simulink model "rhpZeros"  (R2015a)
settings: Solver=ode3  StartTime=0.0  StopTime=10.0  FixedStep=1/200  RelTol=1e-3
undefined symbols (not defined in the file or in its folder): Hinf
libraries: PoliArd x9, simulink x3, dspswit3 x1
settings Model: ExtModeTrigDuration=2  Creator=user  LastModifiedBy=user
settings OptimizationCC: OptimizeModelRefInitCode=on  LifeSpan=1
settings DebuggingCC: UnderspecifiedInitializationDetection=Classic  MergeDetectMultiDrivingBlocksExec=none
settings HardwareCC: ProdLargestAtomicInteger=Long  ProdLargestAtomicFloat=Double  ProdEndianess=LittleEndian  ProdHWDeviceType=ARM Compatible->ARM Cortex
settings RTWCC: SystemTargetFile=realtime.tlc  GenerateMakefile=off  TemplateMakefile=realtime.tmf  Description=Run on Target Hardware  RTWVerbose=off
settings ERTTargetCC: CombineOutputUpdateFcns=off  ExtModeTransport=3  ExtModeMexFile=ext_serial_win32_comm_rtt  ExtModeMexArgs=0 1 9600  ERTSrcFileBannerTemplate=realtime_code_template.cgt  ERTHdrFileBannerTemplate=realtime_code_template.cgt  ERTDataSrcFileTemplate=realtime_code_template.cgt  ERTDataHdrFileTemplate=realtime_code_template.cgt  ERTCustomFileTemplate=realtime_file_process.tlc

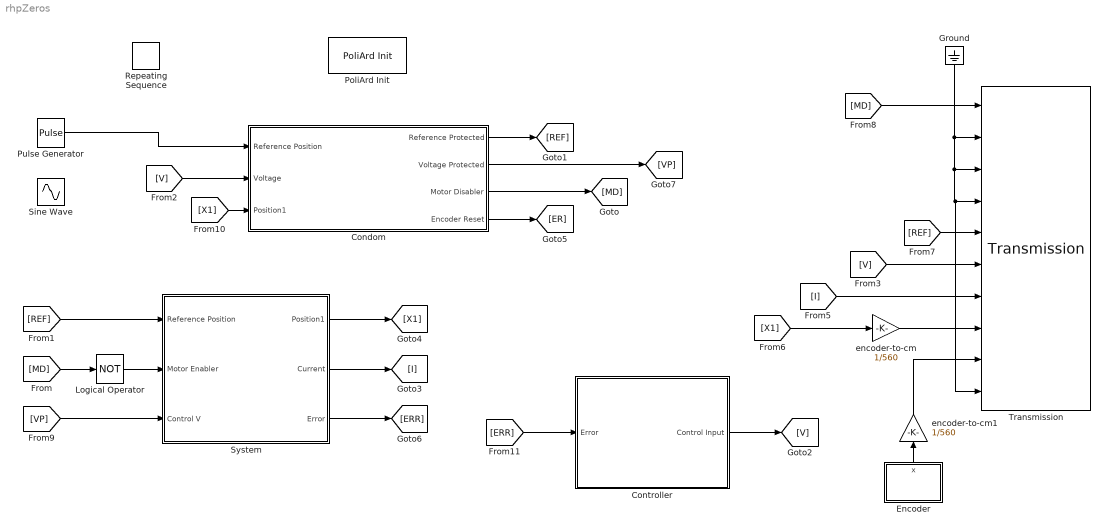
== system rhpZeros ==
  Condom : Subsystem
  Controller : Subsystem
  "Encoder " : Subsystem
  Ground : Ground
  Logical Operator : Logic  Operator=NOT  AllPortsSameDT=off  OutDataTypeStr=boolean
  PoliArd Init : PoliArd/PoliArd Init
  Pulse Generator : DiscretePulseGenerator  PulseType=Time based  Period=10  PulseWidth=50  PhaseDelay=5
  Repeating Sequence : simulink/Sources/Repeating Sequence  rep_seq_t=[0 5]  rep_seq_y=[0 1]
  Sine Wave : Sin  Frequency=2*pi*1  SampleTime=0
  "System " : Subsystem
  Transmission : PoliArd/Transmission  sample_freq=200  sig_to_send=6
  encoder-to-cm : Gain  Gain=1/560
  encoder-to-cm1 : Gain  Gain=1/560
  wires:
  Logical Operator/1 -> "System "/2(Motor Enabler)
  [MD] -> Logical Operator/1
  Condom/1(Reference Protected) -> [REF]
  [REF] -> "System "/1(Reference Position)
  "System "/2(Current) -> [I]
  [V] -> Condom/2(Voltage)
  [V] -> Transmission/6
  [I] -> Transmission/7
  "System "/1(Position1) -> [X1]
  [X1] -> encoder-to-cm/1
  [REF] -> Transmission/5
  [MD] -> Transmission/1
  [VP] -> "System "/3(Control V)
  [X1] -> Condom/3(Position1)
  encoder-to-cm/1 -> Transmission/8
  Controller/1(Control Input) -> [V]
  "System "/3(Error) -> [ERR]
  [ERR] -> Controller/1(Error)
  Condom/2("Voltage Protected ") -> [VP]
  Condom/3(Motor Disabler) -> [MD]
  Condom/4(Encoder Reset) -> [ER]
  Ground/1 -> Transmission/10, Transmission/4, Transmission/3, Transmission/2
  Pulse Generator/1 -> Condom/1(Reference Position)
  "Encoder "/1(x) -> encoder-to-cm1/1
  encoder-to-cm1/1 -> Transmission/9

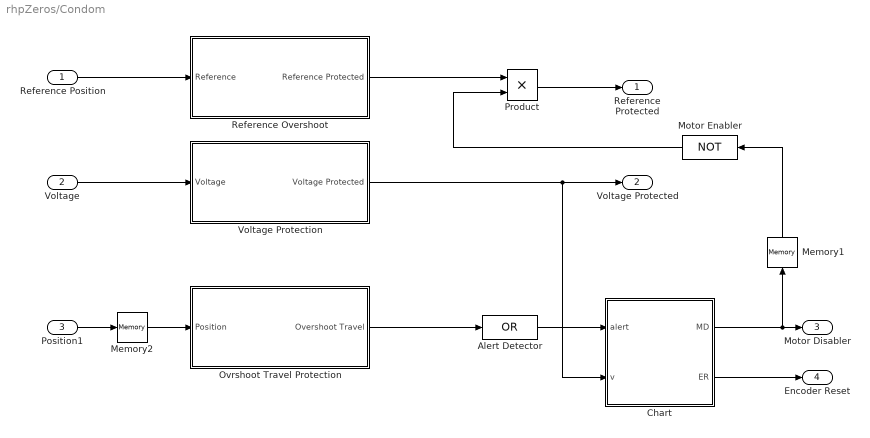
== system rhpZeros/Condom ==
  Reference Position : Inport
  Voltage : Inport  Port=2
  Position1 : Inport  Port=3
  Alert Detector : Logic  Operator=OR  Inputs=1  AllPortsSameDT=off  OutDataTypeStr=boolean
  Chart : Stateflow chart  TreatAsAtomicUnit=on
  Memory1 : Memory
  Memory2 : Memory
  Motor Enabler : Logic  Operator=NOT  Inputs=1  AllPortsSameDT=off  OutDataTypeStr=boolean
  Ovrshoot Travel Protection : Subsystem
  Product : Product
  Reference Overshoot : Subsystem
  Voltage Protection : Subsystem
  Reference Protected : Outport
  "Voltage Protected " : Outport  Port=2
  Motor Disabler : Outport  Port=3
  Encoder Reset : Outport  Port=4
  wires:
  Reference Position/1 -> Reference Overshoot/1("Reference ")
  Memory2/1 -> Ovrshoot Travel Protection/1("Position ")
  Position1/1 -> Memory2/1
  Ovrshoot Travel Protection/1(Overshoot Travel) -> Alert Detector/1
  Alert Detector/1 -> Chart/1(alert)
  Chart/1(MD) -> Motor Disabler/1, Memory1/1
  Chart/2(ER) -> Encoder Reset/1
  Voltage/1 -> Voltage Protection/1("Voltage ")
  Voltage Protection/1(Voltage Protected) -> Chart/2(v), "Voltage Protected "/1
  Product/1 -> Reference Protected/1
  Reference Overshoot/1(Reference Protected) -> Product/1
  Motor Enabler/1 -> Product/2
  Memory1/1 -> Motor Enabler/1

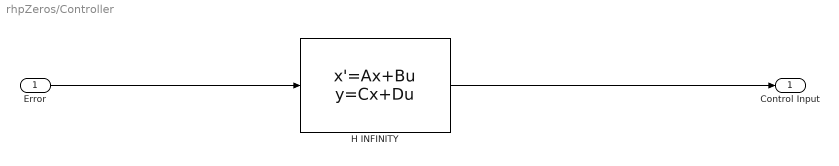
== system rhpZeros/Controller ==
  Error : Inport
  H INFINITY : StateSpace  A=Hinf.A  B=Hinf.B  C=Hinf.C  D=Hinf.D  X0=0
  Control Input : Outport
  wires:
  Error/1 -> H INFINITY/1
  H INFINITY/1 -> Control Input/1

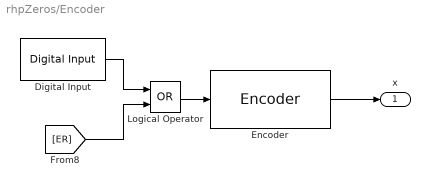
== system rhpZeros/Encoder  ==
  Digital Input : PoliArd/Digital Input  DI_pin=2  DIsample=1/200
  Encoder : PoliArd/Encoder  EncoderID=4  dt_enc=1/200
  Logical Operator : Logic  Operator=OR  AllPortsSameDT=off  OutDataTypeStr=boolean
  x : Outport
  wires:
  Encoder/1 -> x/1
  Digital Input/1 -> Logical Operator/1
  [ER] -> Logical Operator/2
  Logical Operator/1 -> Encoder/1

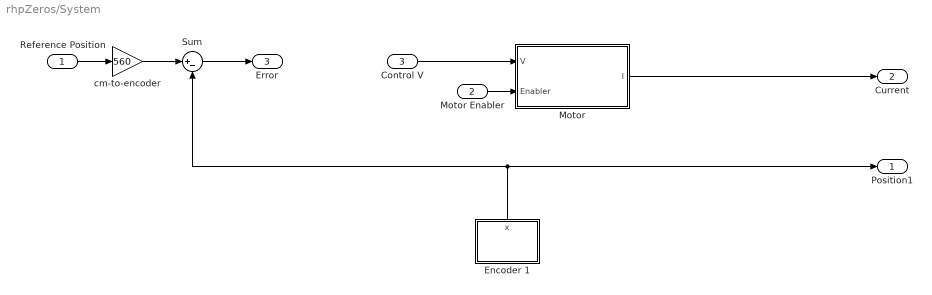
== system rhpZeros/System  ==
  Reference Position : Inport
  Motor Enabler : Inport  Port=2
  Control V : Inport  Port=3
  "Encoder 1 " : Subsystem
  Motor : Subsystem
  Sum : Sum  Inputs=|+-
  cm-to-encoder : Gain  Gain=560
  Position1 : Outport
  Current : Outport  Port=2
  Error : Outport  Port=3
  wires:
  cm-to-encoder/1 -> Sum/1
  Motor/1(I) -> Current/1
  Sum/1 -> Error/1
  Reference Position/1 -> cm-to-encoder/1
  Motor Enabler/1 -> Motor/2(Enabler)
  Control V/1 -> Motor/1(V)
  "Encoder 1 "/1(x) -> Position1/1, Sum/2

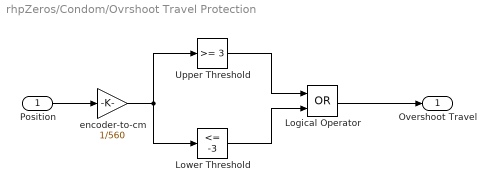
== system rhpZeros/Condom/Ovrshoot Travel Protection ==
  "Position " : Inport
  Logical Operator : Logic  Operator=OR  AllPortsSameDT=off  OutDataTypeStr=boolean
  Lower Threshold : simulink/Logic and Bit Operations/Compare To Constant  relop=<=  const=-3  OutDataTypeStr=boolean
  Upper Threshold : simulink/Logic and Bit Operations/Compare To Constant  relop=>=  const=3  OutDataTypeStr=boolean
  encoder-to-cm : Gain  Gain=1/560
  Overshoot Travel : Outport
  wires:
  Logical Operator/1 -> Overshoot Travel/1
  Lower Threshold/1 -> Logical Operator/2
  Upper Threshold/1 -> Logical Operator/1
  "Position "/1 -> encoder-to-cm/1
  encoder-to-cm/1 -> Lower Threshold/1, Upper Threshold/1

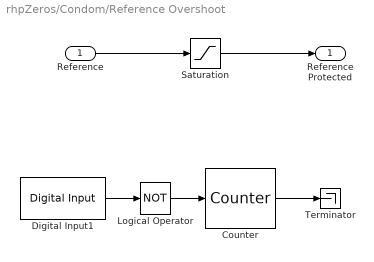
== system rhpZeros/Condom/Reference Overshoot ==
  "Reference " : Inport
  Counter : dspswit3/Counter  Direction=Up  CountEvent=Free running  CounterSize=User defined  MaxCount=10  InitialCount=0  Output=Hit  HitValue=5  ResetInput=on  SamplesPerFrame=1  Ts=1/200  CntDtype=double  HitDtype=Logical
  Digital Input1 : PoliArd/Digital Input  DI_pin=3  DIsample=1/200
  Logical Operator : Logic  Operator=NOT  AllPortsSameDT=off  OutDataTypeStr=boolean
  Saturation : Saturate  UpperLimit=3  LowerLimit=-3
  Terminator : Terminator
  Reference Protected : Outport
  wires:
  Saturation/1 -> Reference Protected/1
  "Reference "/1 -> Saturation/1
  Digital Input1/1 -> Logical Operator/1
  Logical Operator/1 -> Counter/1
  Counter/1 -> Terminator/1

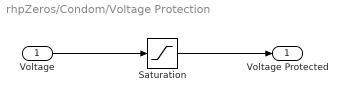
== system rhpZeros/Condom/Voltage Protection ==
  "Voltage " : Inport
  Saturation : Saturate  UpperLimit=5  LowerLimit=-5
  Voltage Protected : Outport
  wires:
  Saturation/1 -> Voltage Protected/1
  "Voltage "/1 -> Saturation/1

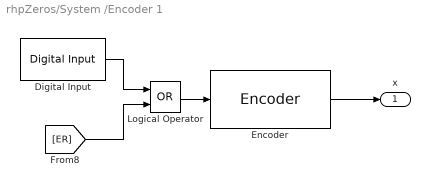
== system rhpZeros/System /Encoder 1  ==
  Digital Input : PoliArd/Digital Input  DI_pin=2  DIsample=1/200
  Encoder : PoliArd/Encoder  EncoderID=1  dt_enc=1/200
  Logical Operator : Logic  Operator=OR  AllPortsSameDT=off  OutDataTypeStr=boolean
  x : Outport
  wires:
  Encoder/1 -> x/1
  Digital Input/1 -> Logical Operator/1
  [ER] -> Logical Operator/2
  Logical Operator/1 -> Encoder/1

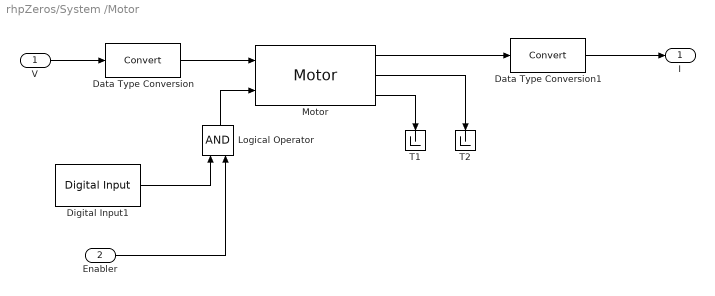
== system rhpZeros/System /Motor ==
  V : Inport
  Enabler : Inport  Port=2
  Data Type Conversion : DataTypeConversion
  Data Type Conversion1 : DataTypeConversion
  Digital Input1 : PoliArd/Digital Input  DI_pin=3  DIsample=1/200
  Logical Operator : Logic  AllPortsSameDT=off  OutDataTypeStr=boolean
  Motor : PoliArd/Motor  MotorID=2  DC_bus_mask=12  dt_mot=1/200
  T1 : Terminator
  T2 : Terminator
  I : Outport
  wires:
  Data Type Conversion/1 -> Motor/1
  V/1 -> Data Type Conversion/1
  Motor/3 -> T1/1
  Motor/2 -> T2/1
  Motor/1 -> Data Type Conversion1/1
  Data Type Conversion1/1 -> I/1
  Enabler/1 -> Logical Operator/2
  Logical Operator/1 -> Motor/2
  Digital Input1/1 -> Logical Operator/1

== stateflow chart rhpZeros/Condom/Chart ==
  state OK
    entry:
    MD=0;
    ER=0;
  state ALERT
    entry:
    MD=1;
    ER=1;
  (default) -> OK
  OK -> ALERT : [alert==1]
  ALERT -> OK : [abs(v)<0.3]
  data: alert input; v input; MD output; ER output
